simulink model "sat"  (R2023b)
settings: Solver=ode15s  StartTime=0.0  StopTime=T_sim  FixedStep=1e-2  RelTol=1e-4
undefined symbols (not defined in the file): A, alpha, B, beta, Bw, C, D, Dw, E, F, leak, N1, nw, Pi_u, Pi_y, Qu, Qy, R, smooth_hard, u_max, u_min, w_const, x0, y_ref
settings Model: Creator=fjako  LastModifiedBy=fjako

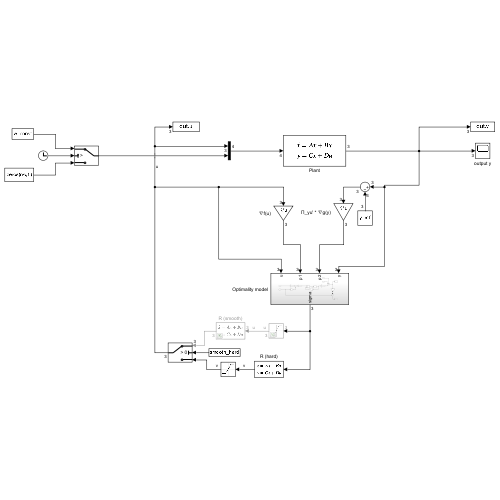
[thumbnail: Simulink's stored preview of the top-level diagram]
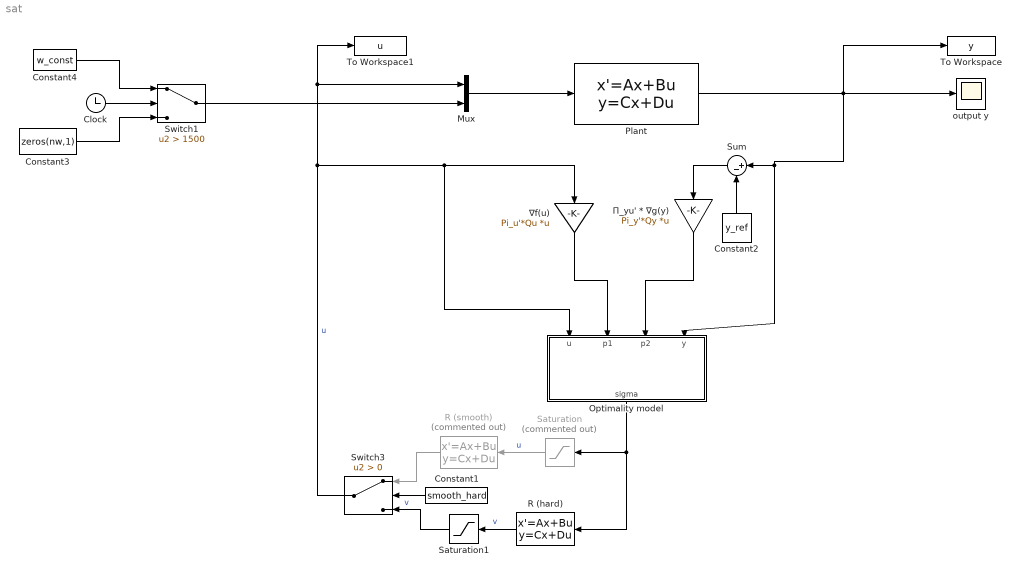
== system sat ==
  Clock : Clock
  Constant1 : Constant  Value=smooth_hard
  Constant2 : Constant  Value=y_ref
  Constant3 : Constant  Value=zeros(nw,1)
  Constant4 : Constant  Value=w_const
  Mux : Mux  Inputs=2
  Optimality model : Subsystem
  Plant : StateSpace  A=A  B=[B Bw]  C=C  D=[D Dw]  InitialCondition=x0
  R (hard) : StateSpace  A=R.A  B=R.B  C=R.C  D=R.D  InitialCondition=0
  R (smooth) : StateSpace  Commented=on  A=R.A  B=R.B  C=R.C  D=R.D  InitialCondition=0
  Saturation : Saturate  Commented=on  UpperLimit=u_max  LowerLimit=u_min
  Saturation1 : Saturate  UpperLimit=u_max  LowerLimit=u_min
  Sum : Sum  Inputs=|+-
  Switch1 : Switch  Criteria=u2 > Threshold  Threshold=1500  SaturateOnIntegerOverflow=off  InputSameDT=off
  Switch3 : Switch  Criteria=u2 > Threshold  SaturateOnIntegerOverflow=off  InputSameDT=off
  To Workspace : ToWorkspace  VariableName=y  SaveFormat=Timeseries  SampleTime=-1
  To Workspace1 : ToWorkspace  VariableName=u  SaveFormat=Timeseries  SampleTime=-1
  output y : Scope
  Π_yu' * ∇g(y) : Gain  Gain=Pi_y'*Qy  Multiplication=Matrix(K*u)
  ∇f(u) : Gain  Gain=Pi_u'*Qu  Multiplication=Matrix(K*u)
  wires:
  Switch1/1 -> Mux/2
  Plant/1 -> Optimality model/4(y), Sum/1, output y/1, To Workspace/1
  Mux/1 -> Plant/1
  Switch3/1 -> Mux/1, To Workspace1/1, Optimality model/1(u), ∇f(u)/1  "u"
  R (hard)/1 -> Saturation1/1  "v"
  Π_yu' * ∇g(y)/1 -> Optimality model/3(p2)
  ∇f(u)/1 -> Optimality model/2(p1)
  Sum/1 -> Π_yu' * ∇g(y)/1
  Constant2/1 -> Sum/2
  Clock/1 -> Switch1/2
  Constant4/1 -> Switch1/1
  Constant3/1 -> Switch1/3
  Saturation/1 -> R (smooth)/1  "u"
  R (smooth)/1 -> Switch3/1
  Constant1/1 -> Switch3/2
  Saturation1/1 -> Switch3/3  "v"
  Optimality model/1(sigma) -> Saturation/1, R (hard)/1

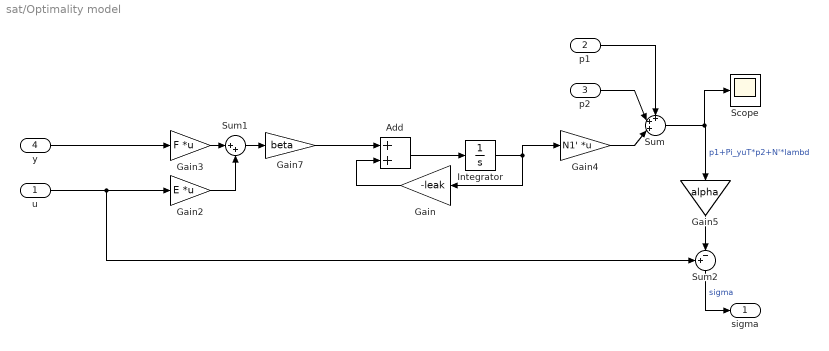
== system sat/Optimality model ==
  u : Inport
  p1 : Inport  Port=2
  p2 : Inport  Port=3
  y : Inport  Port=4
  Add : Sum
  Gain : Gain  Gain=-leak
  Gain2 : Gain  Gain=E  Multiplication=Matrix(K*u)
  Gain3 : Gain  Gain=F  Multiplication=Matrix(K*u)
  Gain4 : Gain  Gain=N1'  Multiplication=Matrix(K*u)
  Gain5 : Gain  Gain=alpha
  Gain7 : Gain  Gain=beta
  Integrator : Integrator
  Scope : Scope
  Sum : Sum  Inputs=+++|
  Sum1 : Sum  Inputs=|++
  Sum2 : Sum  Inputs=+-|
  sigma : Outport
  wires:
  Gain3/1 -> Sum1/1
  Gain2/1 -> Sum1/2
  Sum1/1 -> Gain7/1
  Sum/1 -> Scope/1, Gain5/1  "p1+Pi_yuT*p2+N'*lambd"
  Gain5/1 -> Sum2/2
  y/1 -> Gain3/1
  Sum2/1 -> sigma/1  "sigma"
  u/1 -> Sum2/1, Gain2/1
  Gain4/1 -> Sum/3
  p1/1 -> Sum/1
  p2/1 -> Sum/2
  Gain7/1 -> Add/1
  Add/1 -> Integrator/1
  Integrator/1 -> Gain4/1, Gain/1
  Gain/1 -> Add/2
